simulink model "UpdatedModel16 1"  (R2025b)
settings: Solver=ode23tb  StartTime=0  StopTime=57600  MaxStep=0.005  RelTol=1e-3
settings Model: Creator=charl  LastModifiedBy=Thomas
settings SolverCC: ZeroCrossAlgorithm=Adaptive
settings DataIOCC: DatasetSignalFormat=timetable
settings DebuggingCC: MaskedZcDiagnostic=none  IgnoredZcDiagnostic=none

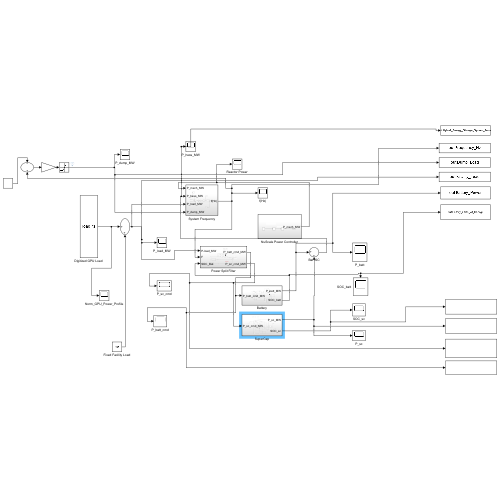
[thumbnail: Simulink's stored preview of the top-level diagram]
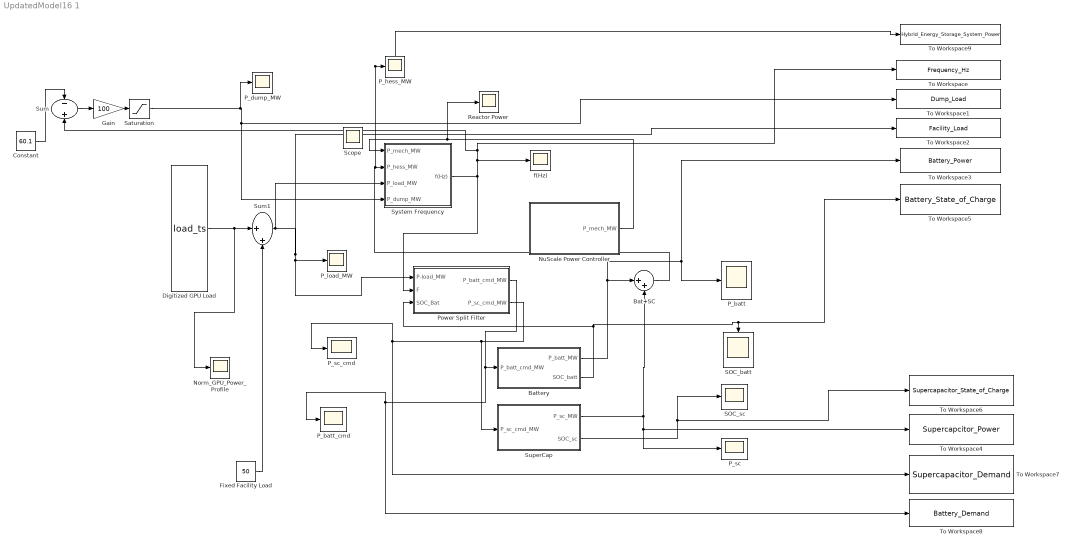
== system UpdatedModel16 1 ==
  Bat+SC : Sum  Inputs=|++
  Battery : Subsystem
  Constant : Constant  Value=60.1
  "Digitized GPU Load " : FromWorkspace  VariableName=load_ts
  Fixed Facility Load : Constant  Value=50
  Gain : Gain  Gain=100
  Norm_GPU_Power_Profile : Scope
      settings: ActiveDisplayYMinimum=7.5678509924416346  ActiveDisplayYMaximum=83.578557138931586  DataLoggingVariableName=ScopeData9
  NuScale Power Controller : Subsystem
  P_batt : Scope
      settings: ActiveDisplayYMinimum=-37.384907164908867  ActiveDisplayYMaximum=19.94300469302301  DataLoggingVariableName=P_batt_MW
  P_batt_cmd : Scope
      settings: ActiveDisplayYMinimum=-187.77485148691687  ActiveDisplayYMaximum=75.99715262684947  DataLoggingVariableName=P_batt_cmd
  P_dump_MW : Scope
      settings: ActiveDisplayYMinimum=6.5603009172756188  ActiveDisplayYMaximum=25.49044457763469  DataLoggingVariableName=P_dump_MW
  P_hess_MW : Scope
      settings: ActiveDisplayYMinimum=-10.620112806422254  ActiveDisplayYMaximum=17.504527906345061  DataLoggingVariableName=P_HESS_MW
  P_load_MW : Scope
      settings: ActiveDisplayYMinimum=58.154484848407179  ActiveDisplayYMaximum=569.112693801637  DataLoggingVariableName=P_load_MW
  P_sc : Scope
      settings: ActiveDisplayYMinimum=-198.52464221560328  ActiveDisplayYMaximum=-106.02414017820828  DataLoggingVariableName=P_sc_MW
  P_sc_cmd : Scope
      settings: ActiveDisplayYMinimum=-8.3010166612799861  ActiveDisplayYMaximum=17.195565288472629  DataLoggingVariableName=P_sc_cmd
  Power Split Filter : Subsystem
  Reactor Power : Scope
      settings: ActiveDisplayYMinimum=149.82124151201739  ActiveDisplayYMaximum=150.0841476543022  DataLoggingVariableName=ScopeData2
  SOC_batt : Scope
      settings: ActiveDisplayYMinimum=-0.29273518191827375  ActiveDisplayYMaximum=1.0471717298948067  DataLoggingVariableName=SOC_batt
  SOC_sc : Scope
      settings: ActiveDisplayYMinimum=0.11776806010766516  ActiveDisplayYMaximum=0.73168131364842448  DataLoggingVariableName=SOC_sc
  Saturation : Saturate  UpperLimit=250  LowerLimit=0
  Sum : Sum  Inputs=-+
  Sum1 : Sum  Inputs=|++
  SuperCap : Subsystem
  System Frequency : Subsystem
  To Workspace : ToWorkspace  VariableName=Frequency_Hz  SaveFormat=Timeseries  SampleTime=-1
  To Workspace1 : ToWorkspace  VariableName=Dump_Load  SaveFormat=Timeseries  SampleTime=-1
  To Workspace2 : ToWorkspace  VariableName=Facility_Load  SaveFormat=Timeseries  SampleTime=-1
  To Workspace3 : ToWorkspace  VariableName=Battery_Power  SaveFormat=Timeseries  SampleTime=-1
  To Workspace4 : ToWorkspace  VariableName=Supercapcitor_Power  SaveFormat=Timeseries  SampleTime=-1
  To Workspace5 : ToWorkspace  VariableName=Battery_State_of_Charge  SaveFormat=Timeseries  SampleTime=-1
  To Workspace6 : ToWorkspace  VariableName=Supercapacitor_State_of_Charge  SaveFormat=Timeseries  SampleTime=-1
  To Workspace7 : ToWorkspace  VariableName=Supercapacitor_Demand  SaveFormat=Timeseries  SampleTime=-1
  To Workspace8 : ToWorkspace  VariableName=Battery_Demand  SaveFormat=Timeseries  SampleTime=-1
  To Workspace9 : ToWorkspace  VariableName=Hybrid_Energy_Storage_System_Power  SaveFormat=Timeseries  SampleTime=-1
  f(Hz) : Scope
      settings: ActiveDisplayYMinimum=43.509673055268742  ActiveDisplayYMaximum=72.466557603230314  DataLoggingVariableName=f_Hz
  Scope : Scope
      settings: ActiveDisplayYMinimum=-1  ActiveDisplayYMaximum=1
  wires:
  "Digitized GPU Load "/1 -> Norm_GPU_Power_Profile/1, Sum1/1
  System Frequency/1(f(Hz)) -> Sum/2, To Workspace/1, f(Hz)/1, Power Split Filter/2(F)
  NuScale Power Controller/1(P_mech_MW) -> Reactor Power/1, System Frequency/1(P_mech_MW)
  Power Split Filter/1(P_batt_cmd_MW) -> To Workspace8/1, P_batt_cmd/1, Battery/1(P_batt_cmd_MW)
  Battery/2(SOC_batt) -> To Workspace5/1, SOC_batt/1, Power Split Filter/3(SOC_Bat)
  Power Split Filter/2(P_sc_cmd_MW) -> P_sc_cmd/1, To Workspace7/1, SuperCap/1(P_sc_cmd_MW)
  Battery/1(P_batt_MW) -> P_batt/1, To Workspace3/1, Bat+SC/1
  SuperCap/1(P_sc_MW) -> Bat+SC/2, P_sc/1, To Workspace4/1
  Bat+SC/1 -> System Frequency/2(P_hess_MW), To Workspace9/1, P_hess_MW/1
  Fixed Facility Load/1 -> Sum1/2
  SuperCap/2(SOC_sc) -> SOC_sc/1, To Workspace6/1
  Sum1/1 -> Power Split Filter/1(P-load_MW), P_load_MW/1, To Workspace2/1, System Frequency/3(P_load_MW)
  Sum/1 -> Gain/1
  Constant/1 -> Sum/1
  Gain/1 -> Saturation/1
  Saturation/1 -> P_dump_MW/1, To Workspace1/1, System Frequency/4(P_dump_MW)

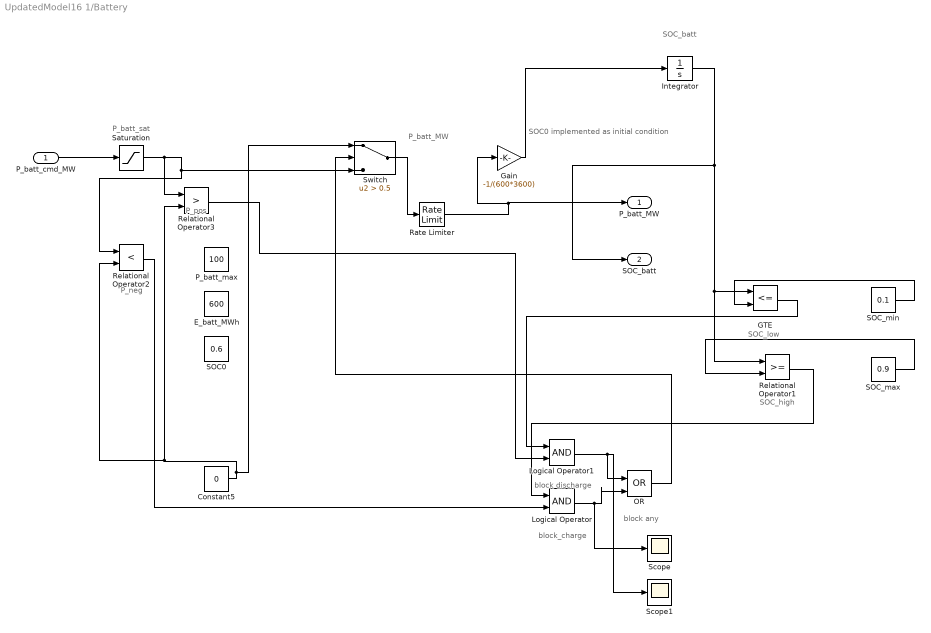
== system UpdatedModel16 1/Battery ==
  note: block any
  note: block_charge
  note: block discharge
  note: SOC_high
  note: SOC_low
  note: P_neg
  note: P_pos
  note: SOC_batt
  note: P_batt_MW
  note: P_batt_sat
  note: SOC0 implemented as initial condition
  P_batt_cmd_MW : Inport
  Constant5 : Constant  Value=0
  E_batt_MWh : Constant  Value=600
  GTE : RelationalOperator  Operator=<=  OutDataTypeStr=boolean  RndMeth=Simplest  InputSameDT=off
  Gain : Gain  Gain=-1/(600*3600)
  Integrator : Integrator  InitialCondition=0.5
  Logical Operator : Logic  AllPortsSameDT=off  OutDataTypeStr=boolean
  Logical Operator1 : Logic  AllPortsSameDT=off  OutDataTypeStr=boolean
  OR : Logic  Operator=OR  IconShape=distinctive  AllPortsSameDT=off  OutDataTypeStr=boolean
  P_batt_max : Constant  Value=100
  Rate Limiter : RateLimiter  RisingSlewLimit=50  FallingSlewLimit=-50  SampleTimeMode=inherited
  Relational Operator1 : RelationalOperator  OutDataTypeStr=boolean  RndMeth=Simplest  InputSameDT=off
  Relational Operator2 : RelationalOperator  Operator=<  OutDataTypeStr=boolean  RndMeth=Simplest  InputSameDT=off
  Relational Operator3 : RelationalOperator  Operator=>  OutDataTypeStr=boolean  RndMeth=Simplest  InputSameDT=off
  SOC0 : Constant  Value=0.6
  SOC_max : Constant  Value=0.9
  SOC_min : Constant  Value=0.1
  Saturation : Saturate  UpperLimit=100  LowerLimit=-100
  Scope : Scope
      settings: ActiveDisplayYMinimum=-13.085244769910002  ActiveDisplayYMaximum=17.941319549660328  DataLoggingVariableName=ScopeData5
  Scope1 : Scope
      settings: ActiveDisplayYMinimum=-1  ActiveDisplayYMaximum=1  DataLoggingVariableName=ScopeData6
  Switch : Switch  Criteria=u2 > Threshold  Threshold=0.5  SaturateOnIntegerOverflow=off  InputSameDT=off
  P_batt_MW : Outport
  SOC_batt : Outport  Port=2
  wires:
  P_batt_cmd_MW/1 -> Saturation/1
  Constant5/1 -> Switch/1, Relational Operator2/2, Relational Operator3/2
  Gain/1 -> Integrator/1
  Integrator/1 -> GTE/1, Relational Operator1/1, SOC_batt/1
  Saturation/1 -> Switch/3, Relational Operator2/1, Relational Operator3/1
  Relational Operator3/1 -> Logical Operator1/2
  Relational Operator2/1 -> Logical Operator/2
  Logical Operator1/1 -> Scope1/1, OR/1
  Logical Operator/1 -> Scope/1, OR/2
  Rate Limiter/1 -> Gain/1, P_batt_MW/1
  Switch/1 -> Rate Limiter/1
  SOC_min/1 -> GTE/2
  SOC_max/1 -> Relational Operator1/2
  OR/1 -> Switch/2
  Relational Operator1/1 -> Logical Operator/1
  GTE/1 -> Logical Operator1/1

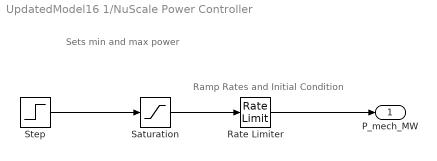
== system UpdatedModel16 1/NuScale Power Controller ==
  note: Ramp Rates and Initial Condition
  note: Sets min and max power
  Rate Limiter : RateLimiter  RisingSlewLimit=0.385  FallingSlewLimit=-0.385  SampleTimeMode=inherited  InitialCondition=300  LinearizeAsGain=off
  Saturation : Saturate  UpperLimit=308  LowerLimit=60
  Step : Step  Time=28760  Before=305  After=150  SampleTime=0
  P_mech_MW : Outport
  wires:
  Rate Limiter/1 -> P_mech_MW/1
  Step/1 -> Saturation/1
  Saturation/1 -> Rate Limiter/1

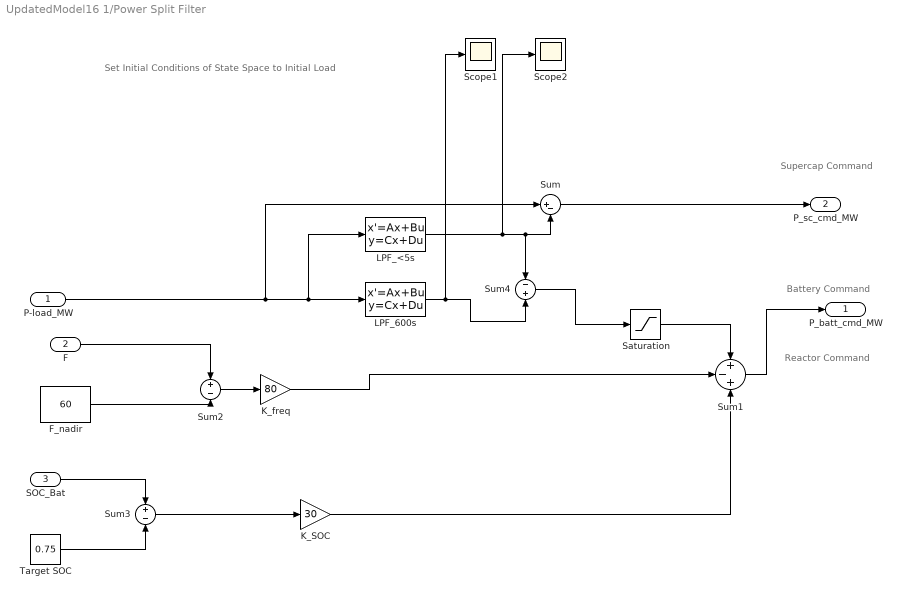
== system UpdatedModel16 1/Power Split Filter ==
  note: Set Initial Conditions of State Space to Initial Load
  note: Reactor Command
  note: Battery Command
  note: Supercap Command
  P-load_MW : Inport
  F : Inport  Port=2
  SOC_Bat : Inport  Port=3
  F_nadir : Constant  Value=60
  K_SOC : Gain  Gain=30
  K_freq : Gain  Gain=80
  LPF_600s : StateSpace  A=-1/900  B=1/900  D=0  InitialCondition=280
  LPF_<5s : StateSpace  A=-0.2  B=0.2  D=0  InitialCondition=280
  Saturation : Saturate  UpperLimit=25  LowerLimit=-25
  Scope1 : Scope
      settings: ActiveDisplayYMinimum=49.062612418746049  ActiveDisplayYMaximum=145.81639543994109  DataLoggingVariableName=ScopeData3
  Scope2 : Scope
      settings: ActiveDisplayYMinimum=59.667836185063258  ActiveDisplayYMaximum=63.141494099133709  DataLoggingVariableName=ScopeData4
  Sum : Sum  Inputs=|+-
  Sum1 : Sum  Inputs=+-+
  Sum2 : Sum  Inputs=+-
  Sum3 : Sum  Inputs=+-
  Sum4 : Sum  Inputs=-+
  Target SOC : Constant  Value=0.75
  P_batt_cmd_MW : Outport  OutMin=-15  OutMax=15
  P_sc_cmd_MW : Outport  Port=2  OutMin=-10  OutMax=10
  wires:
  P-load_MW/1 -> Sum/1, LPF_<5s/1, LPF_600s/1
  Sum/1 -> P_sc_cmd_MW/1
  LPF_<5s/1 -> Sum4/1, Sum/2, Scope2/1
  Sum1/1 -> P_batt_cmd_MW/1
  LPF_600s/1 -> Sum4/2, Scope1/1
  F/1 -> Sum2/1
  F_nadir/1 -> Sum2/2
  Sum2/1 -> K_freq/1
  K_freq/1 -> Sum1/2
  SOC_Bat/1 -> Sum3/1
  Target SOC/1 -> Sum3/2
  Sum3/1 -> K_SOC/1
  ? -> ?
  K_SOC/1 -> Sum1/3
  Sum4/1 -> Saturation/1
  Saturation/1 -> Sum1/1

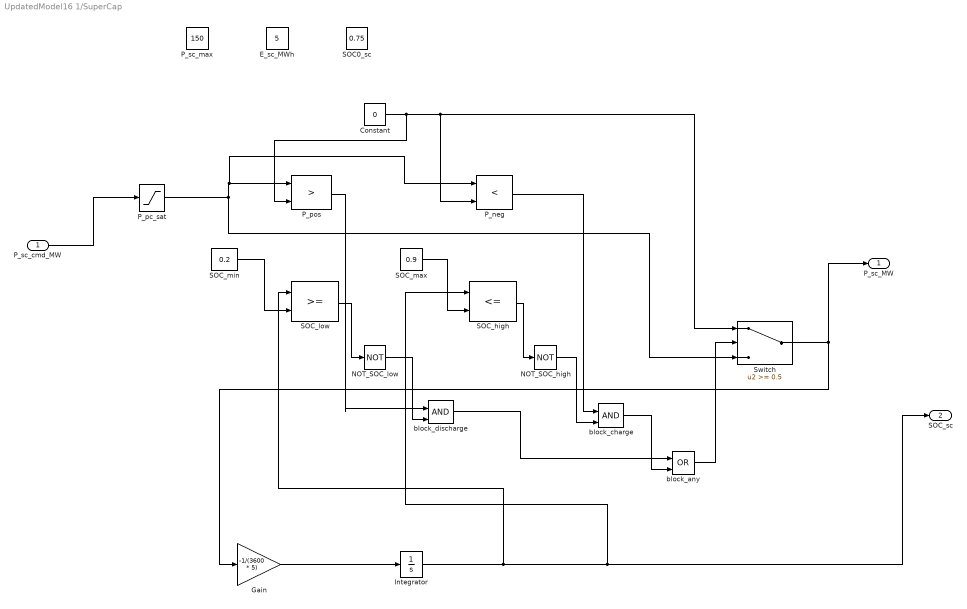
== system UpdatedModel16 1/SuperCap ==
  P_sc_cmd_MW : Inport
  Constant : Constant  Value=0
  E_sc_MWh : Constant  Value=5
  Gain : Gain  Gain=-1/(3600 * 5)
  Integrator : Integrator  InitialCondition=0.5
  NOT_SOC_high : Logic  Operator=NOT  IconShape=distinctive  AllPortsSameDT=off  OutDataTypeStr=boolean
  NOT_SOC_low : Logic  Operator=NOT  IconShape=distinctive  AllPortsSameDT=off  OutDataTypeStr=boolean
  P_neg : RelationalOperator  Operator=<  OutDataTypeStr=boolean  RndMeth=Simplest  InputSameDT=off
  P_pc_sat : Saturate  UpperLimit=150  LowerLimit=-150
  P_pos : RelationalOperator  Operator=>  OutDataTypeStr=boolean  RndMeth=Simplest  InputSameDT=off
  P_sc_max : Constant  Value=150
  SOC0_sc : Constant  Value=0.75
  SOC_high : RelationalOperator  Operator=<=  OutDataTypeStr=boolean  RndMeth=Simplest  InputSameDT=off
  SOC_low : RelationalOperator  OutDataTypeStr=boolean  RndMeth=Simplest  InputSameDT=off
  SOC_max : Constant  Value=0.9
  SOC_min : Constant  Value=0.2
  Switch : Switch  Threshold=0.5  SaturateOnIntegerOverflow=off  InputSameDT=off
  block_any : Logic  Operator=OR  IconShape=distinctive  AllPortsSameDT=off  OutDataTypeStr=boolean
  block_charge : Logic  IconShape=distinctive  AllPortsSameDT=off  OutDataTypeStr=boolean
  block_discharge : Logic  IconShape=distinctive  AllPortsSameDT=off  OutDataTypeStr=boolean
  P_sc_MW : Outport
  SOC_sc : Outport  Port=2
  wires:
  P_sc_cmd_MW/1 -> P_pc_sat/1
  P_pc_sat/1 -> Switch/3, P_neg/1, P_pos/1
  Constant/1 -> P_pos/2, Switch/1, P_neg/2
  SOC_max/1 -> SOC_high/2
  SOC_min/1 -> SOC_low/2
  SOC_low/1 -> NOT_SOC_low/1
  SOC_high/1 -> NOT_SOC_high/1
  P_pos/1 -> block_discharge/1
  NOT_SOC_low/1 -> block_discharge/2
  P_neg/1 -> block_charge/1
  NOT_SOC_high/1 -> block_charge/2
  block_charge/1 -> block_any/2
  block_discharge/1 -> block_any/1
  block_any/1 -> Switch/2
  Gain/1 -> Integrator/1
  Integrator/1 -> SOC_low/1, SOC_high/1, SOC_sc/1
  Switch/1 -> Gain/1, P_sc_MW/1

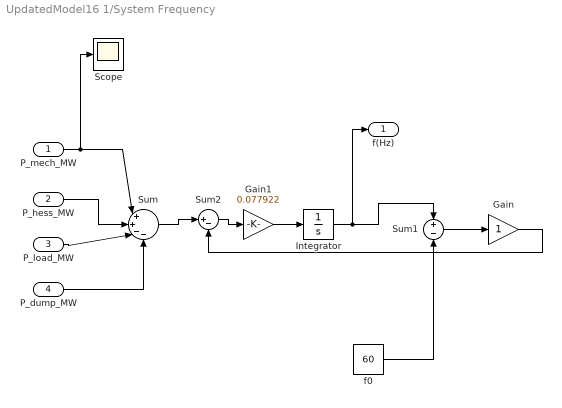
== system UpdatedModel16 1/System Frequency ==
  P_mech_MW : Inport
  P_hess_MW : Inport  Port=2
  P_load_MW : Inport  Port=3
  P_dump_MW : Inport  Port=4
  Gain : Gain
  Gain1 : Gain  Gain=0.077922
  Integrator : Integrator  InitialCondition=60
  Scope : Scope
      settings: ActiveDisplayYMinimum=-1  ActiveDisplayYMaximum=1
  Sum : Sum  Inputs=|++--
  Sum1 : Sum  Inputs=+-
  Sum2 : Sum  Inputs=|+-
  f0 : Constant  Value=60
  f(Hz) : Outport
  wires:
  f0/1 -> Sum1/2
  Sum1/1 -> Gain/1
  P_mech_MW/1 -> Scope/1, Sum/1
  P_hess_MW/1 -> Sum/2
  P_load_MW/1 -> Sum/3
  P_dump_MW/1 -> Sum/4
  Sum/1 -> Sum2/1
  Gain/1 -> Sum2/2
  Sum2/1 -> Gain1/1
  Gain1/1 -> Integrator/1
  Integrator/1 -> f(Hz)/1, Sum1/1
